simulink model "moonlander_fuzzy2"  (R2024b)
settings: Solver=ode2  StartTime=0.0  StopTime=inf  FixedStep=0.1  RelTol=1e-3
values from neighbouring files (symbols this model uses):
  gamma = 6.6743e-11    [pramaters.m]    (also in rl_init_parameters.m)
  h0 = 10e3    (= 10000)    [pramaters.m]    (also in rl_init_parameters.m)
  M = 7.346e22    (= 7.346e+22)    [pramaters.m]    (also in rl_init_parameters.m)
  m0 = m0_sol + m0_fuel    (= 10000)    [pramaters.m]    (also in rl_init_parameters.m)
  m0_fuel = 8e3    (= 8000)    [pramaters.m]    (also in rl_init_parameters.m)
  mdmax = Pmax/2500    (= 18)    [pramaters.m]    (also in rl_init_parameters.m)
  Pmax = 45e3    (= 45000)    [pramaters.m]    (also in rl_init_parameters.m)
  R = 3474e3/2    (= 1737000)    [pramaters.m]    (also in rl_init_parameters.m)
libraries: simulink x3, fuzblock x2
settings Model: Creator=grote_w  LastModifiedBy=grote_w
settings RTWCC: GPUComputeCapability=3.5

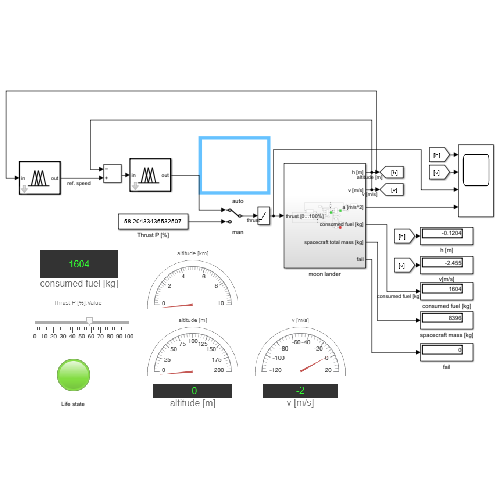
[thumbnail: Simulink's stored preview of the top-level diagram]
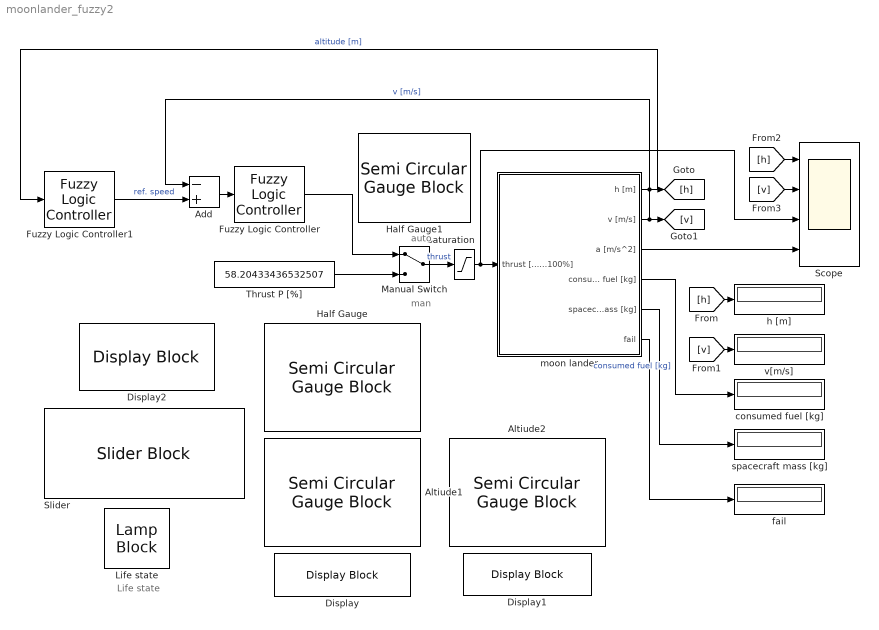
== system moonlander_fuzzy2 ==
  note: Life state
  note: man
  note: auto
  Add : Sum  Inputs=-+
  Altiude1 : SemiCircularGaugeBlock  ScaleMax=200
  Altiude2 : SemiCircularGaugeBlock  ScaleMin=-120  ScaleMax=20
  Display : DisplayBlock  LabelPosition=Bottom  Format=Integer  Transparency=1
  Display1 : DisplayBlock  LabelPosition=Bottom  Format=Integer  Transparency=1
  Display2 : DisplayBlock  LabelPosition=Bottom  Format=Integer  Transparency=1
  Fuzzy Logic Controller : fuzblock/Fuzzy Logic  Controller  FIS='thrust.fis'  OutputSampleNumber=101  DataType=double  FuzzifiedInputs=off  RuleFiringStrengths=off  RuleOutputs=off  AggregatedOutputs=off  SimulateUsing=Interpreted execution  OutOfRangeInputValueMessage=warning  NoRuleFiredMessage=warning  EmptyOutputFuzzySetMessage=warning
  Fuzzy Logic Controller1 : fuzblock/Fuzzy Logic  Controller  FIS='refspeed.fis'  OutputSampleNumber=101  DataType=double  FuzzifiedInputs=off  RuleFiringStrengths=off  RuleOutputs=off  AggregatedOutputs=off  SimulateUsing=Interpreted execution  OutOfRangeInputValueMessage=warning  NoRuleFiredMessage=warning  EmptyOutputFuzzySetMessage=warning
  Half Gauge : SemiCircularGaugeBlock  ScaleMax=10
  Half Gauge1 : SemiCircularGaugeBlock
  Life state : LampBlock  LabelPosition=Hide
  Manual Switch : ManualSwitch
  Saturation : Saturate  UpperLimit=100  LowerLimit=0
  Scope : Scope  NumInputPorts=4
  Slider : SliderBlock
  Thrust P [%] : Constant  Value=58.20433436532507
  consumed fuel [kg] : Display
  fail : Display
  h [m] : Display
  moon lander : Subsystem
  spacecraft mass [kg] : Display
  v[m/s] : Display
  wires:
  Thrust P [%]/1 -> Manual Switch/2
  Manual Switch/1 -> Saturation/1  "thrust"
  moon lander/4(consumed fuel [kg]) -> consumed fuel [kg]/1  "consumed fuel [kg]"
  moon lander/5(spacecraft total mass [kg]) -> spacecraft mass [kg]/1
  moon lander/3(a [m/s^2]) -> Scope/4
  moon lander/6(fail) -> fail/1
  moon lander/1(h [m]) -> Fuzzy Logic Controller1/1, [h]  "altitude [m]"
  moon lander/2(v [m/s]) -> Add/1, [v]  "v [m/s]"
  [h] -> h [m]/1
  [v] -> v[m/s]/1
  [h] -> Scope/1
  [v] -> Scope/2
  Saturation/1 -> moon lander/1(thrust [0...100%]), Scope/3
  Fuzzy Logic Controller/1 -> Manual Switch/1
  Add/1 -> Fuzzy Logic Controller/1
  Fuzzy Logic Controller1/1 -> Add/2  "ref. speed"

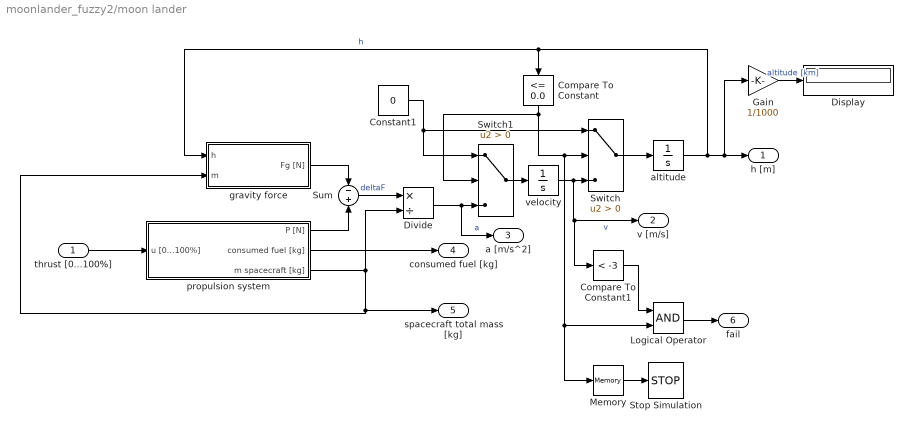
== system moonlander_fuzzy2/moon lander ==
  thrust [0...100%] : Inport
  Compare To Constant : simulink/Logic and Bit Operations/Compare To Constant  relop=<=  const=0.0  OutDataTypeStr=boolean
  Compare To Constant1 : simulink/Logic and Bit Operations/Compare To Constant  relop=<  const=-3  OutDataTypeStr=boolean
  Constant1 : Constant  Value=0
  Display : Display
  Divide : Product  Inputs=*/
  Gain : Gain  Gain=1/1000
  Logical Operator : Logic  AllPortsSameDT=off  OutDataTypeStr=boolean
  Memory : Memory
  Stop Simulation : Stop
  Sum : Sum  Inputs=-+
  Switch : Switch  Criteria=u2 > Threshold  SaturateOnIntegerOverflow=off  InputSameDT=off
  Switch1 : Switch  Criteria=u2 > Threshold  SaturateOnIntegerOverflow=off  InputSameDT=off
  altitude : Integrator  InitialCondition=h0
  gravity force : Subsystem
  propulsion system : Subsystem
  velocity : Integrator
  h [m] : Outport
  v [m/s] : Outport  Port=2
  a [m/s^2] : Outport  Port=3
  consumed fuel [kg] : Outport  Port=4
  spacecraft total mass [kg] : Outport  Port=5
  fail : Outport  Port=6
  wires:
  Constant1/1 -> Switch/1, Switch1/1
  velocity/1 -> Compare To Constant1/1, v [m/s]/1, Switch/3  "v"
  Compare To Constant/1 -> Switch1/2, Memory/1, Logical Operator/2, Switch/2
  Sum/1 -> Divide/1  "deltaF"
  altitude/1 -> Gain/1, h [m]/1, Compare To Constant/1, gravity force/1(h)  "h"
  gravity force/1(Fg [N]) -> Sum/1
  propulsion system/3(m spacecraft [kg]) -> gravity force/2(m), spacecraft total mass [kg]/1, Divide/2
  Switch/1 -> altitude/1
  Switch1/1 -> velocity/1
  propulsion system/2(consumed fuel [kg]) -> consumed fuel [kg]/1
  propulsion system/1(P [N]) -> Sum/2
  Divide/1 -> a [m/s^2]/1, Switch1/3  "a"
  thrust [0...100%]/1 -> propulsion system/1(u [0...100%])
  Compare To Constant1/1 -> Logical Operator/1
  Logical Operator/1 -> fail/1
  Memory/1 -> Stop Simulation/1
  Gain/1 -> Display/1  "altitude [km]"

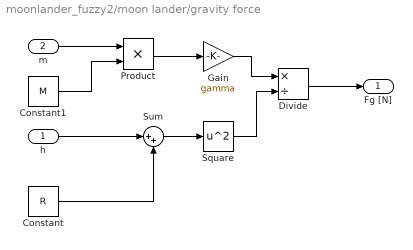
== system moonlander_fuzzy2/moon lander/gravity force ==
  h : Inport
  m : Inport  Port=2
  Constant : Constant  Value=R
  Constant1 : Constant  Value=M
  Divide : Product  Inputs=*/
  Gain : Gain  Gain=gamma
  Product : Product
  Square : Math  Operator=square
  Sum : Sum  Inputs=|++
  Fg [N] : Outport
  wires:
  h/1 -> Sum/1
  Constant/1 -> Sum/2
  Constant1/1 -> Product/2
  m/1 -> Product/1
  Product/1 -> Gain/1
  Sum/1 -> Square/1
  Gain/1 -> Divide/1
  Square/1 -> Divide/2
  Divide/1 -> Fg [N]/1

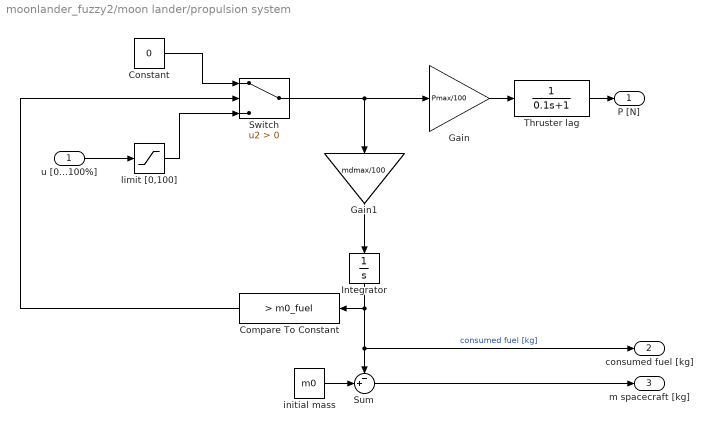
== system moonlander_fuzzy2/moon lander/propulsion system ==
  u [0...100%] : Inport
  Compare To Constant : simulink/Logic and Bit Operations/Compare To Constant  relop=>  const=m0_fuel  OutDataTypeStr=boolean
  Constant : Constant  Value=0
  Gain : Gain  Gain=Pmax/100
  Gain1 : Gain  Gain=mdmax/100
  Integrator : Integrator  UpperSaturationLimit=m0_fuel  LowerSaturationLimit=0
  Sum : Sum  Inputs=-+|
  Switch : Switch  Criteria=u2 > Threshold  SaturateOnIntegerOverflow=off  InputSameDT=off
  Thruster lag : TransferFcn  Denominator=[0.1 1]
  initial mass : Constant  Value=m0
  limit [0,100] : Saturate  UpperLimit=100  LowerLimit=0
  P [N] : Outport
  consumed fuel [kg] : Outport  Port=2
  m spacecraft [kg] : Outport  Port=3
  wires:
  Gain/1 -> Thruster lag/1
  Switch/1 -> Gain/1, Gain1/1
  Thruster lag/1 -> P [N]/1
  initial mass/1 -> Sum/2
  Sum/1 -> m spacecraft [kg]/1
  Integrator/1 -> Compare To Constant/1, consumed fuel [kg]/1, Sum/1  "consumed fuel [kg]"
  Gain1/1 -> Integrator/1
  Compare To Constant/1 -> Switch/2
  u [0...100%]/1 -> limit [0,100]/1
  Constant/1 -> Switch/1
  limit [0,100]/1 -> Switch/3
